simulink model "craneest"  (R2022b)
settings: Solver=ode45  StartTime=0.0  StopTime=50  RelTol=1e-3  EnableMultiTasking=on
values from neighbouring files (symbols this model uses):
  F = [0 1 0 0;   0 -(b/M+mp^2*l^2*b/(A*M^2)) mp^2*l^2*g/(A*M) 0;  0 0 0 1;  0 mp*l*b/(A*M) -mp*g*l/A 0]    [initcrane.m]
  G = [0; 1/M+mp^2*l^2/(A*M^2); 0 ; -mp*l/(A*M)]    [initcrane.m]
  H = eye(4)    [initcrane.m]
  H1 = [1 0 0 0; 0 0 1 0]    [initcrane.m]
  J = zeros(4,1)    [initcrane.m]
  K = acker(F,G,2*[-0.5 -0.5 -1 -1])    [initcrane.m]
  L = LL'    [initcrane.m]
  x0 = [];end    [craneanim.m]    (also in initcrane.m = [35 0 0 0])
libraries: simulink x1
settings Model: Creator=beghi  LastModifiedBy=meme
settings SolverCC: AlgebraicLoopSolver=TrustRegion
settings DataIOCC: LimitDataPoints=on  SaveFormat=Array  SignalLoggingSaveFormat=ModelDataLogs  ReturnWorkspaceOutputs=off  SignalLoggingName=sigsOut
settings OptimizationCC: ExpressionDepthLimit=2147483647  InitFltsAndDblsToZero=on  LifeSpan=inf
settings DebuggingCC: SaveWithParameterizedLinksMsg=none  UnderspecifiedInitializationDetection=Classic  MergeDetectMultiDrivingBlocksExec=none  SignalResolutionControl=TryResolveAllWithWarning  MultiTaskDSMMsg=warning  MultiTaskCondExecSysMsg=none  FcnCallInpInsideContextMsg=warning  UnconnectedInputMsg=warning  UnconnectedOutputMsg=warning  UnconnectedLineMsg=warning  StateNameClashWarn=warning  SFUnexpectedBacktrackingDiag=warning  SFNoUnconditionalDefaultTransitionDiag=warning  SFExecutionAtInitializationDiag=none  SFMachineParentedDataDiag=warning  ArithmeticOperatorsInVariantConditions=warning
settings HardwareCC: ProdBitPerPointer=32  ProdBitPerSizeT=32  ProdBitPerPtrDiffT=32  ProdLargestAtomicFloat=None  ProdIntDivRoundTo=Undefined  ProdEndianess=Unspecified  ProdWordSize=32  ProdHWDeviceType=32-bit Generic  TargetUnknown=on
settings ModelReferenceCC: EnableRefExpFcnMdlSchedulingChecks=on  PropagateSignalLabelsOutOfModel=off
settings SFSimCC: SimUseLocalCustomCode=off  CustomCodeUndefinedFunction=UseInterfaceOnly
settings RTWCC: RTWUseLocalCustomCode=off
settings CodeAppCC: StateflowObjectComments=on
settings GRTTargetCC: TargetFcnLib=ansi_tfl_tmw.mat  TargetLangStandard=C89/C90 (ANSI)  ModelReferenceCompliant=off  CombineOutputUpdateFcns=off  MatFileLogging=off  GRTInterface=on
settings ConfigComp: CovMetricSettings=dw  CovSaveCumulativeToWorkspaceVar=on  CovSaveSingleToWorkspaceVar=on  CovExternalEMLEnable=off

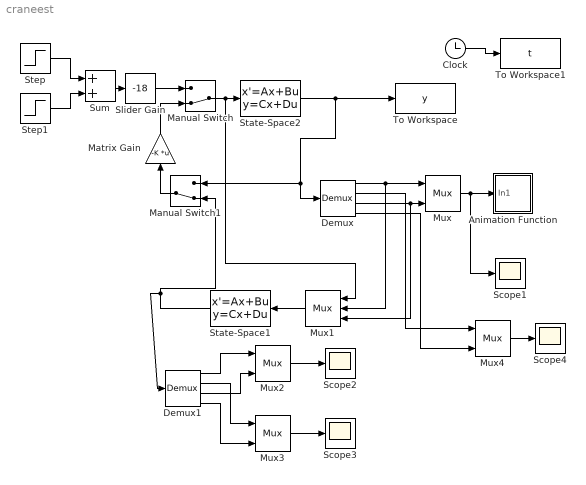
== system craneest ==
  Animation Function : Subsystem  mask(Animation Block){ts=0.05}
      mask prompts: ts "Sample time:"
      mask Display: plot([.1,.9],[.9,.9],[.5,.2],[.9,.25],[.475,.475,.525,.525,.475],[.875,.925,.925,.875,.875])
  Clock : Clock
  Demux : Demux
      settings: DisplayOption=none
  Demux1 : Demux
      settings: DisplayOption=none
  Manual Switch : ManualSwitch  CurrentSetting=0
  Manual Switch1 : ManualSwitch  CurrentSetting=0
  Matrix Gain : Gain  Gain=-K  Multiplication=Matrix(K*u)  SaturateOnIntegerOverflow=on  OutDataTypeStr=Inherit: Same as input  ParamDataTypeStr=Inherit: Same as input
  Mux{,2..4} (4 alike) : Mux  Inputs=2
  Mux1 : Mux  Inputs=3
  Scope{1..4} (4 alike) : Scope
  Slider Gain : simulink/Math Operations/Slider Gain  gain=-18  low=-20  high=20
  State-Space1 : StateSpace  A=F-L*H1  B=[G L]  C=eye(4)  D=zeros(4,3)  InitialCondition=zeros(4,1)
  State-Space2 : StateSpace  A=F  B=G  C=H  D=J  InitialCondition=x0
  Step : Step
  Step1 : Step  Time=5  After=-1
  Sum : Sum  InputSameDT=on  SaturateOnIntegerOverflow=on  OutDataTypeStr=Inherit: Same as first input
  To Workspace : ToWorkspace  VariableName=y  SampleTime=-1
  To Workspace1 : ToWorkspace  VariableName=t  SampleTime=-1
  wires:
  Step/1 -> Sum/1
  Step1/1 -> Sum/2
  Sum/1 -> Slider Gain/1
  State-Space2/1 -> To Workspace/1, Demux/1, Manual Switch1/1
  Clock/1 -> To Workspace1/1
  Mux/1 -> Animation Function/1(In1), Scope1/1
  Demux/1 -> Mux/1, Mux1/2
  Demux/3 -> Mux/2, Mux1/3
  Manual Switch/1 -> Mux1/1, State-Space2/1
  Slider Gain/1 -> Manual Switch/1
  Mux1/1 -> State-Space1/1
  State-Space1/1 -> Manual Switch1/2, Demux1/1
  Manual Switch1/1 -> Matrix Gain/1
  Matrix Gain/1 -> Manual Switch/2
  Demux1/1 -> Mux2/1
  Demux1/3 -> Mux2/2
  Mux2/1 -> Scope2/1
  Mux3/1 -> Scope3/1
  Demux1/2 -> Mux3/1
  Demux1/4 -> Mux3/2
  Demux/2 -> Mux4/1
  Demux/4 -> Mux4/2
  Mux4/1 -> Scope4/1

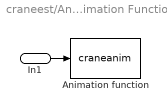
== system craneest/Animation Function ==
  In1 : Inport
  Animation function : S-Function  FunctionName=craneanim  Parameters=ts  SFunctionDeploymentMode=off  EnableBusSupport=off
      settings: DeleteFcn=if ~isempty(findobj('type','figure','name','simppend Animation'));close('simppend Animation'); end;
  wires:
  In1/1 -> Animation function/1
